simulink model "Exercitiul2_1"  (R2016a)
settings: Solver=VariableStepAuto  StartTime=0.0  StopTime=50  RelTol=1e-3
undefined symbols (not defined in the file): entitySys, m, n, ShowPriority
settings Model: Creator=Cristina  LastModifiedBy=Cristina

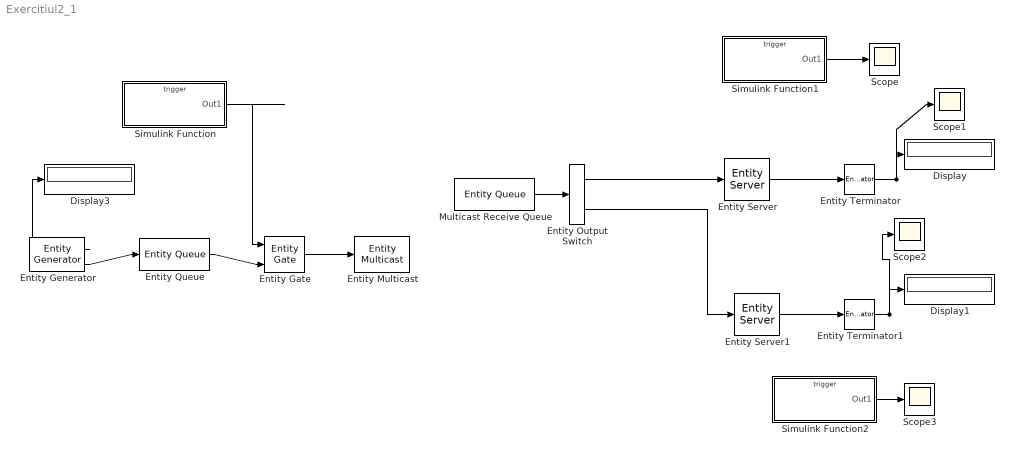
== system Exercitiul2_1 ==
  Display : Display
  Display1 : Display
  Display3 : Display
  Entity Output Switch : EntityOutputSwitch  InputPortMessageModes=m  OutputPortMessageModes=m,m  SwitchingCriterion=Equiprobable  SwitchAttributeName=Attribute1
  Entity Gate : EntityGate  InputPortMessageModes=m,m  OutputPortMessageModes=m
  Entity Generator : EntityGenerator  OutputPortMessageModes=n,m  TimeSource=MATLAB action  IntergenerationTimeAction=dt = exprnd(0.1);  GenerateAction=|  AttributeName=CheckinTime  AttributeInitialValue=1 + 1 * rand  NumberEntitiesDeparted=on  EntityType=Structured  EntityTypeName=Entity  EntityPriority=1
      | persistent number;
      | number = rand;
      | if (number < 0.33)
      |     entitySys.priority = 1;
      | else if (number < 0.66)
      |         entitySys.priority = 2;
      | else entitySys.priority = 3;
      | end
      settings: OutputPortMap=o0,o3
  Entity Multicast : EntityMulticast  InputPortMessageModes=m  MulticastTag=Tag
  Entity Queue : EntityQueue  InputPortMessageModes=m  OutputPortMessageModes=m  EntryAction=|
      | persistent nEntered
      | if(isempty(nEntered))
      |     nEntered=0;
      | end
      | nEntered = nEntered+1;
      | if(nEntered > 4)
      |     OpenGate(nEntered);
      | end
      | entitySys.priority = round(1 + 2 * rand);
      settings: OutputPortMap=o5
  Entity Server : EntityServer  InputPortMessageModes=m  OutputPortMessageModes=m  Capacity=1  ServiceTimeSource=Attribute  ServiceTimeAttributeName=CheckinTime
  Entity Server1 : EntityServer  InputPortMessageModes=m  OutputPortMessageModes=m  Capacity=1  ServiceTimeSource=Attribute  ServiceTimeAttributeName=CheckinTime
  Entity Terminator : EntityTerminator  InputPortMessageModes=m  EntryAction=ShowPriority(entitySys.priority);  NumberEntitiesArrived=on
      settings: OutputPortMap=o0
  Entity Terminator1 : EntityTerminator  InputPortMessageModes=m  EntryAction=ShowPriority(entitySys.priority);  NumberEntitiesArrived=on
      settings: OutputPortMap=o0
  Multicast Receive Queue : EntityQueue  OutputPortMessageModes=m  QueueType=Priority  PrioritySource=entitySys.priority  SortingDirection=Descending  EntityArrivalSource=Multicast  MulticastTag=Tag
      settings: OutputPortMap=o5
  Scope{,1..3} (4 alike) : Scope
  Simulink Function : Subsystem  TreatAsAtomicUnit=on
  Simulink Function1 : Subsystem  TreatAsAtomicUnit=on
  Simulink Function2 : Subsystem  TreatAsAtomicUnit=on
  wires:
  Entity Generator/2 -> Entity Queue/1
  Entity Queue/1 -> Entity Gate/2
  Entity Gate/1 -> Entity Multicast/1
  Entity Server/1 -> Entity Terminator/1
  Entity Server1/1 -> Entity Terminator1/1
  Simulink Function/1(Out1) -> Entity Gate/1
  Entity Terminator/1 -> Scope1/1, Display/1
  Entity Terminator1/1 -> Scope2/1, Display1/1
  Entity Generator/1 -> Display3/1
  Simulink Function1/1(Out1) -> Scope/1
  Multicast Receive Queue/1 -> Entity Output Switch/1
  Entity Output Switch/1 -> Entity Server/1
  Entity Output Switch/2 -> Entity Server1/1
  Simulink Function2/1(Out1) -> Scope3/1

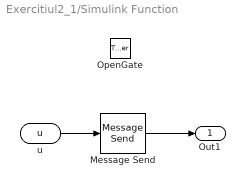
== system Exercitiul2_1/Simulink Function ==
  OpenGate : TriggerPort  TriggerType=function-call  IsSimulinkFunction=on  FunctionName=OpenGate  VariantControl=Variant
  Message Send : MessageSend  OutputPortMessageModes=m
      settings: InputPortMap=u1
  u : ArgIn  DisableCoverage=on  ArgumentName=u
  Out1 : Outport
  wires:
  u/1 -> Message Send/1
  Message Send/1 -> Out1/1

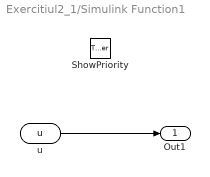
== system Exercitiul2_1/Simulink Function1 ==
  ShowPriority : TriggerPort  TriggerType=function-call  IsSimulinkFunction=on  FunctionName=ShowPriority  VariantControl=Variant
  u : ArgIn  DisableCoverage=on  ArgumentName=u
  Out1 : Outport
  wires:
  u/1 -> Out1/1

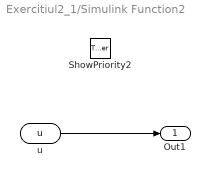
== system Exercitiul2_1/Simulink Function2 ==
  ShowPriority2 : TriggerPort  TriggerType=function-call  IsSimulinkFunction=on  FunctionName=ShowPriority2  VariantControl=Variant
  u : ArgIn  DisableCoverage=on  ArgumentName=u
  Out1 : Outport
  wires:
  u/1 -> Out1/1
